simulink model "SFPPB_RL_simulate"  (R2025b)
settings: Solver=ode4  StartTime=0.0  StopTime=30  FixedStep=0.001  RelTol=1e-3
settings Model: Creator=31586  LastModifiedBy=31586

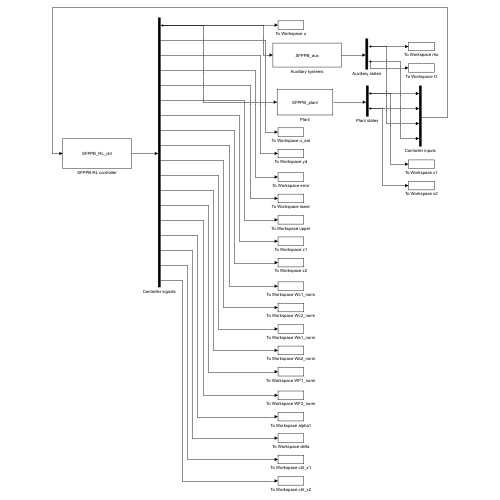
[thumbnail: Simulink's stored preview of the top-level diagram]
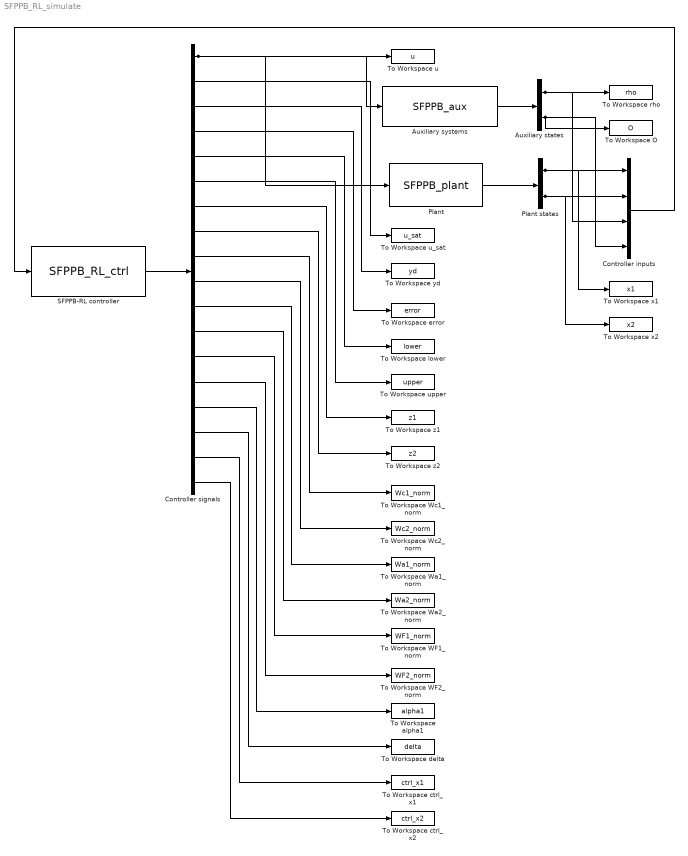
== system SFPPB_RL_simulate ==
  Auxiliary states : Demux  Outputs=2
  Auxiliary systems : S-Function  FunctionName=SFPPB_aux  SFunctionDeploymentMode=off  EnableBusSupport=off
  Controller inputs : Mux
  Controller signals : Demux  Outputs=18
  Plant : S-Function  FunctionName=SFPPB_plant  SFunctionDeploymentMode=off  EnableBusSupport=off
  Plant states : Demux  Outputs=2
  SFPPB-RL controller : S-Function  FunctionName=SFPPB_RL_ctrl  SFunctionDeploymentMode=off  EnableBusSupport=off
  To Workspace O : ToWorkspace  VariableName=O  SaveFormat=Timeseries  SampleTime=-1
  To Workspace WF1_norm : ToWorkspace  VariableName=WF1_norm  SaveFormat=Timeseries  SampleTime=-1
  To Workspace WF2_norm : ToWorkspace  VariableName=WF2_norm  SaveFormat=Timeseries  SampleTime=-1
  To Workspace Wa1_norm : ToWorkspace  VariableName=Wa1_norm  SaveFormat=Timeseries  SampleTime=-1
  To Workspace Wa2_norm : ToWorkspace  VariableName=Wa2_norm  SaveFormat=Timeseries  SampleTime=-1
  To Workspace Wc1_norm : ToWorkspace  VariableName=Wc1_norm  SaveFormat=Timeseries  SampleTime=-1
  To Workspace Wc2_norm : ToWorkspace  VariableName=Wc2_norm  SaveFormat=Timeseries  SampleTime=-1
  To Workspace alpha1 : ToWorkspace  VariableName=alpha1  SaveFormat=Timeseries  SampleTime=-1
  To Workspace ctrl_x1 : ToWorkspace  VariableName=ctrl_x1  SaveFormat=Timeseries  SampleTime=-1
  To Workspace ctrl_x2 : ToWorkspace  VariableName=ctrl_x2  SaveFormat=Timeseries  SampleTime=-1
  To Workspace delta : ToWorkspace  VariableName=delta  SaveFormat=Timeseries  SampleTime=-1
  To Workspace error : ToWorkspace  VariableName=error  SaveFormat=Timeseries  SampleTime=-1
  To Workspace lower : ToWorkspace  VariableName=lower  SaveFormat=Timeseries  SampleTime=-1
  To Workspace rho : ToWorkspace  VariableName=rho  SaveFormat=Timeseries  SampleTime=-1
  To Workspace u : ToWorkspace  VariableName=u  SaveFormat=Timeseries  SampleTime=-1
  To Workspace u_sat : ToWorkspace  VariableName=u_sat  SaveFormat=Timeseries  SampleTime=-1
  To Workspace upper : ToWorkspace  VariableName=upper  SaveFormat=Timeseries  SampleTime=-1
  To Workspace x1 : ToWorkspace  VariableName=x1  SaveFormat=Timeseries  SampleTime=-1
  To Workspace x2 : ToWorkspace  VariableName=x2  SaveFormat=Timeseries  SampleTime=-1
  To Workspace yd : ToWorkspace  VariableName=yd  SaveFormat=Timeseries  SampleTime=-1
  To Workspace z1 : ToWorkspace  VariableName=z1  SaveFormat=Timeseries  SampleTime=-1
  To Workspace z2 : ToWorkspace  VariableName=z2  SaveFormat=Timeseries  SampleTime=-1
  wires:
  Controller signals/1 -> Plant/1, Auxiliary systems/1, To Workspace u/1
  SFPPB-RL controller/1 -> Controller signals/1
  Controller signals/9 -> To Workspace Wc1_norm/1
  Controller signals/3 -> To Workspace yd/1
  Controller signals/5 -> To Workspace lower/1
  Controller signals/7 -> To Workspace z1/1
  Controller signals/8 -> To Workspace z2/1
  Controller signals/2 -> To Workspace u_sat/1
  Controller signals/4 -> To Workspace error/1
  Controller signals/6 -> To Workspace upper/1
  Controller signals/16 -> To Workspace delta/1
  Controller signals/14 -> To Workspace WF2_norm/1
  Controller signals/12 -> To Workspace Wa2_norm/1
  Controller signals/10 -> To Workspace Wc2_norm/1
  Controller signals/17 -> To Workspace ctrl_x1/1
  Controller signals/15 -> To Workspace alpha1/1
  Controller signals/13 -> To Workspace WF1_norm/1
  Controller signals/11 -> To Workspace Wa1_norm/1
  Auxiliary states/1 -> Controller inputs/3, To Workspace rho/1
  Controller signals/18 -> To Workspace ctrl_x2/1
  Auxiliary states/2 -> Controller inputs/4, To Workspace O/1
  Auxiliary systems/1 -> Auxiliary states/1
  Plant/1 -> Plant states/1
  Plant states/1 -> Controller inputs/1, To Workspace x1/1
  Plant states/2 -> Controller inputs/2, To Workspace x2/1
  Controller inputs/1 -> SFPPB-RL controller/1
